simulink model "DigitBreak"  (R2014a)
settings: Solver=FixedStepDiscrete  StartTime=0.0  StopTime=2  FixedStep=1/8000  RelTol=1e-3
undefined symbols (not defined in the file): i
libraries: dspmtrx3 x7, dspsrcs4 x7, simulink x2, dspstat3 x1
settings Model: Creator=Dolby  LastModifiedBy=100432553
settings DataIOCC: SaveOutput=off  SaveTime=off
settings DebuggingCC: UnderspecifiedInitializationDetection=Classic  StateNameClashWarn=warning

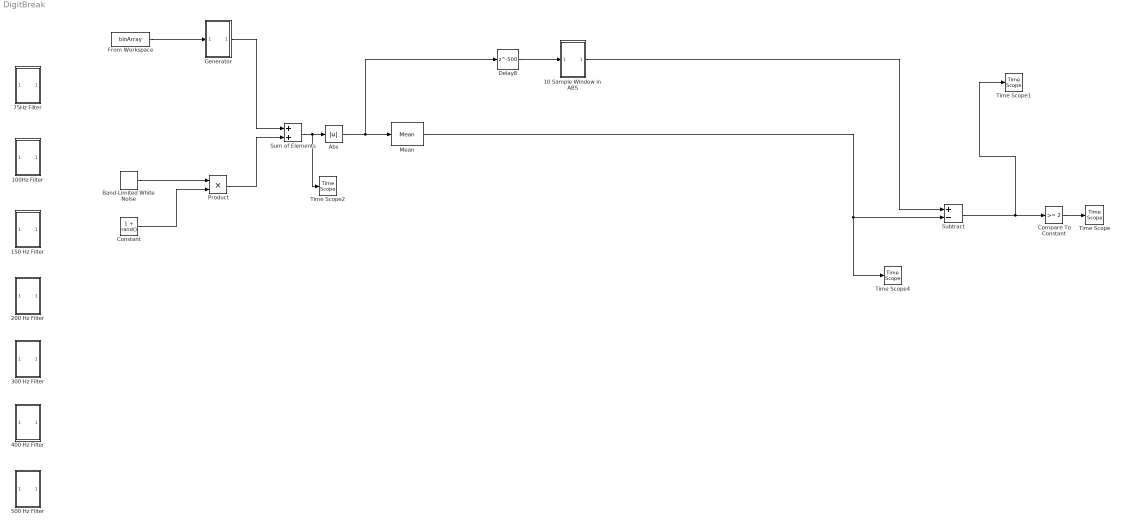
== system DigitBreak ==
  10 Sample Window in ABS : Subsystem
  100Hz Filter : Subsystem
  150 Hz Filter : Subsystem
  200 Hz Filter : Subsystem
  "300 Hz Filter " : Subsystem
  400 Hz Filter : Subsystem
  500 Hz Filter : Subsystem
  75Hz Filter : Subsystem
  Abs : Abs
  Band-Limited White Noise : simulink/Sources/Band-Limited White Noise  Cov=[0.0000001]  Ts=1/8000  seed=[1]
  Compare To Constant : simulink/Logic and Bit Operations/Compare To Constant  relop=>=  const=2  OutDataTypeStr=boolean
  Constant : Constant  Value=1 + rand()
  Delay8 : Delay  DelayLength=500  InitialCondition=0
  From Workspace : FromWorkspace  VariableName=binArray
  Generator : Subsystem
  Mean : dspstat3/Mean  run=on  reset_popup=None  InputProcessing=Columns as channels (frame based)  directionMode=Each column  dimension=1  treatSBRowAsCol=on  roiEnable=off  roiType=Rectangles  roiPortion=Entire ROI  roiOutput=Individual statistics for each ROI  roiFlag=off  outputDataTypeStr=Inherit: Same as accumulator  outputLastDataTypeStr=Inherit: Same as accumulator  outputMin=[]  outputMax=[]  roundingMode=Floor  overflowMode=off
  Product : Product
  Subtract : Sum  Inputs=+-
  Sum of Elements : Sum
  Time Scope{,1..2,4} (4 alike) : TimeScope  DefaultConfigurationName=spbscopes.TimeScopeBlockCfg
  wires:
  From Workspace/1 -> Generator/1(In1)
  Band-Limited White Noise/1 -> Product/1
  Constant/1 -> Product/2
  Sum of Elements/1 -> Time Scope2/1, Abs/1
  Product/1 -> Sum of Elements/2
  Abs/1 -> Mean/1, Delay8/1
  Compare To Constant/1 -> Time Scope/1
  Generator/1(Out1) -> Sum of Elements/1
  Delay8/1 -> 10 Sample Window in ABS/1(In1)
  Mean/1 -> Subtract/2, Time Scope4/1
  Subtract/1 -> Time Scope1/1, Compare To Constant/1
  10 Sample Window in ABS/1(Out1) -> Subtract/1

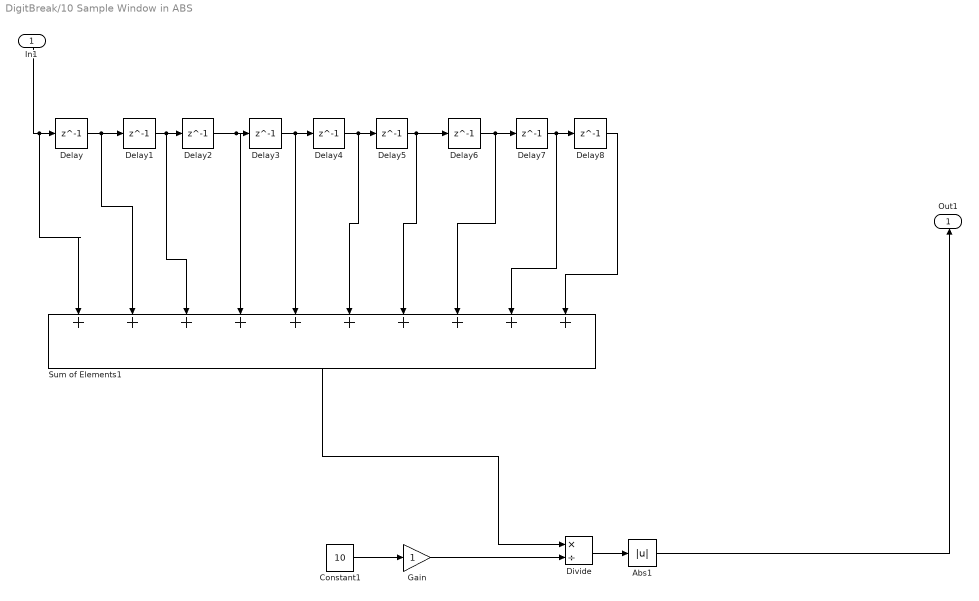
== system DigitBreak/10 Sample Window in ABS ==
  In1 : Inport
  Abs1 : Abs
  Constant1 : Constant  Value=10
  Delay{,1..8} (9 alike) : Delay  DelayLength=1  InitialCondition=0
  Divide : Product  Inputs=*/
  Gain : Gain
  Sum of Elements1 : Sum  Inputs=++++++++++
  Out1 : Outport
  wires:
  Delay4/1 -> Sum of Elements1/6, Delay5/1
  Constant1/1 -> Gain/1
  Divide/1 -> Abs1/1
  Abs1/1 -> Out1/1
  Delay2/1 -> Sum of Elements1/4, Delay3/1
  Delay1/1 -> Sum of Elements1/3, Delay2/1
  Delay/1 -> Sum of Elements1/2, Delay1/1
  Delay3/1 -> Sum of Elements1/5, Delay4/1
  In1/1 -> Delay/1, Sum of Elements1/1
  Gain/1 -> Divide/2
  Sum of Elements1/1 -> Divide/1
  Delay8/1 -> Sum of Elements1/10
  Delay6/1 -> Sum of Elements1/8, Delay7/1
  Delay7/1 -> Sum of Elements1/9, Delay8/1
  Delay5/1 -> Sum of Elements1/7, Delay6/1

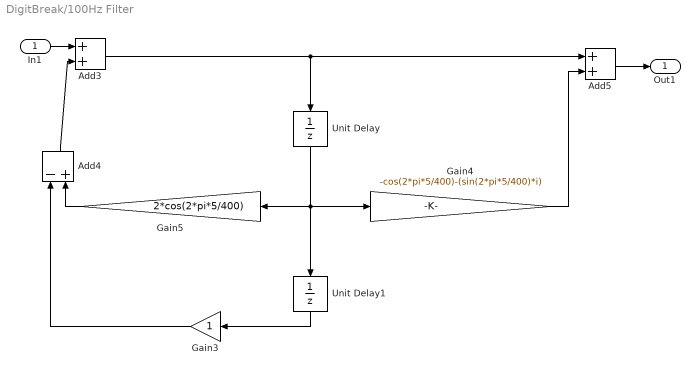
== system DigitBreak/100Hz Filter ==
  In1 : Inport
  Add3 : Sum
  Add4 : Sum  Inputs=-+
  Add5 : Sum
  Gain3 : Gain
  Gain4 : Gain  Gain=-cos(2*pi*5/400)-(sin(2*pi*5/400)*i)
  Gain5 : Gain  Gain=2*cos(2*pi*5/400)
  Unit Delay : UnitDelay  SampleTime=-1
  Unit Delay1 : UnitDelay  SampleTime=-1
  Out1 : Outport
  wires:
  In1/1 -> Add3/1
  Add4/1 -> Add3/2
  Gain3/1 -> Add4/1
  Add3/1 -> Unit Delay/1, Add5/1
  Add5/1 -> Out1/1
  Gain5/1 -> Add4/2
  Gain4/1 -> Add5/2
  Unit Delay1/1 -> Gain3/1
  Unit Delay/1 -> Gain4/1, Unit Delay1/1, Gain5/1

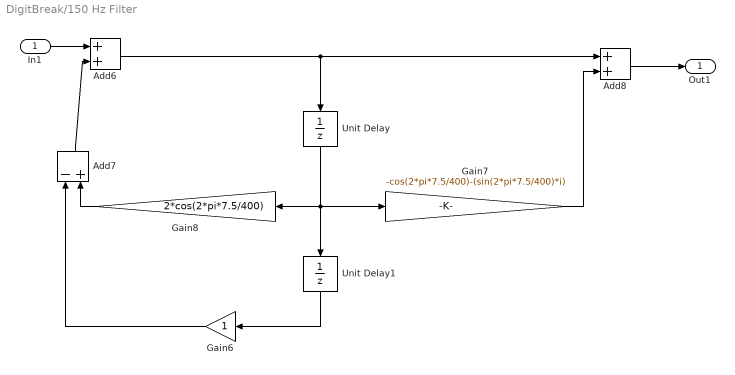
== system DigitBreak/150 Hz Filter ==
  In1 : Inport
  Add6 : Sum
  Add7 : Sum  Inputs=-+
  Add8 : Sum
  Gain6 : Gain
  Gain7 : Gain  Gain=-cos(2*pi*7.5/400)-(sin(2*pi*7.5/400)*i)
  Gain8 : Gain  Gain=2*cos(2*pi*7.5/400)
  Unit Delay : UnitDelay  SampleTime=-1
  Unit Delay1 : UnitDelay  SampleTime=-1
  Out1 : Outport
  wires:
  In1/1 -> Add6/1
  Gain7/1 -> Add8/2
  Add8/1 -> Out1/1
  Gain8/1 -> Add7/2
  Add7/1 -> Add6/2
  Gain6/1 -> Add7/1
  Add6/1 -> Unit Delay/1, Add8/1
  Unit Delay1/1 -> Gain6/1
  Unit Delay/1 -> Gain7/1, Unit Delay1/1, Gain8/1

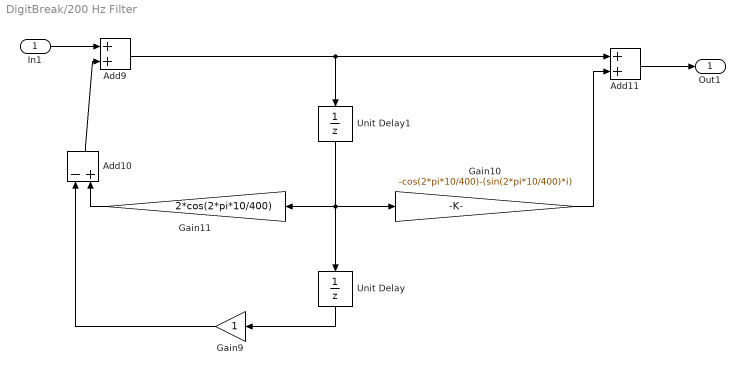
== system DigitBreak/200 Hz Filter ==
  In1 : Inport
  Add10 : Sum  Inputs=-+
  Add11 : Sum
  Add9 : Sum
  Gain10 : Gain  Gain=-cos(2*pi*10/400)-(sin(2*pi*10/400)*i)
  Gain11 : Gain  Gain=2*cos(2*pi*10/400)
  Gain9 : Gain
  Unit Delay : UnitDelay  SampleTime=-1
  Unit Delay1 : UnitDelay  SampleTime=-1
  Out1 : Outport
  wires:
  Gain10/1 -> Add11/2
  Unit Delay1/1 -> Unit Delay/1, Gain10/1, Gain11/1
  Gain9/1 -> Add10/1
  Add10/1 -> Add9/2
  Unit Delay/1 -> Gain9/1
  Add11/1 -> Out1/1
  Add9/1 -> Unit Delay1/1, Add11/1
  Gain11/1 -> Add10/2
  In1/1 -> Add9/1

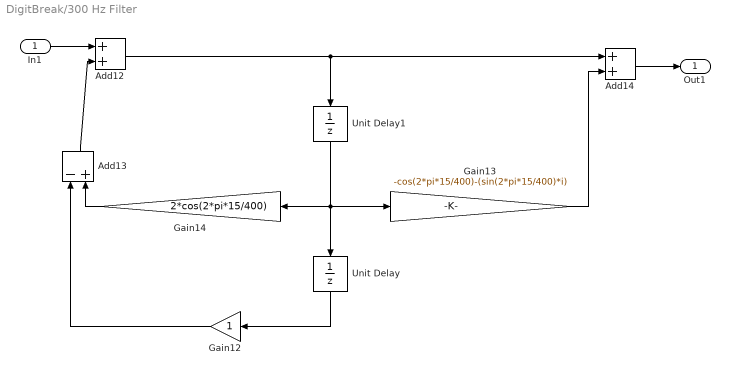
== system DigitBreak/300 Hz Filter  ==
  In1 : Inport
  Add12 : Sum
  Add13 : Sum  Inputs=-+
  Add14 : Sum
  Gain12 : Gain
  Gain13 : Gain  Gain=-cos(2*pi*15/400)-(sin(2*pi*15/400)*i)
  Gain14 : Gain  Gain=2*cos(2*pi*15/400)
  Unit Delay : UnitDelay  SampleTime=-1
  Unit Delay1 : UnitDelay  SampleTime=-1
  Out1 : Outport
  wires:
  Add14/1 -> Out1/1
  Add12/1 -> Unit Delay1/1, Add14/1
  Gain12/1 -> Add13/1
  Unit Delay1/1 -> Unit Delay/1, Gain13/1, Gain14/1
  Add13/1 -> Add12/2
  Gain13/1 -> Add14/2
  Unit Delay/1 -> Gain12/1
  Gain14/1 -> Add13/2
  In1/1 -> Add12/1

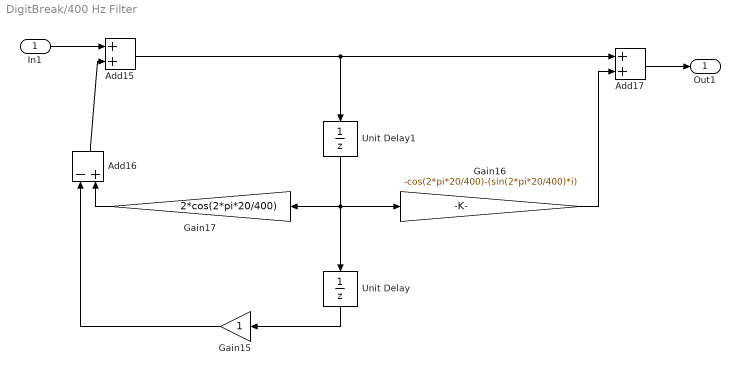
== system DigitBreak/400 Hz Filter ==
  In1 : Inport
  Add15 : Sum
  Add16 : Sum  Inputs=-+
  Add17 : Sum
  Gain15 : Gain
  Gain16 : Gain  Gain=-cos(2*pi*20/400)-(sin(2*pi*20/400)*i)
  Gain17 : Gain  Gain=2*cos(2*pi*20/400)
  Unit Delay : UnitDelay  SampleTime=-1
  Unit Delay1 : UnitDelay  SampleTime=-1
  Out1 : Outport
  wires:
  Gain17/1 -> Add16/2
  Add16/1 -> Add15/2
  Add15/1 -> Unit Delay1/1, Add17/1
  Gain15/1 -> Add16/1
  Unit Delay1/1 -> Gain16/1, Gain17/1, Unit Delay/1
  Gain16/1 -> Add17/2
  Add17/1 -> Out1/1
  Unit Delay/1 -> Gain15/1
  In1/1 -> Add15/1

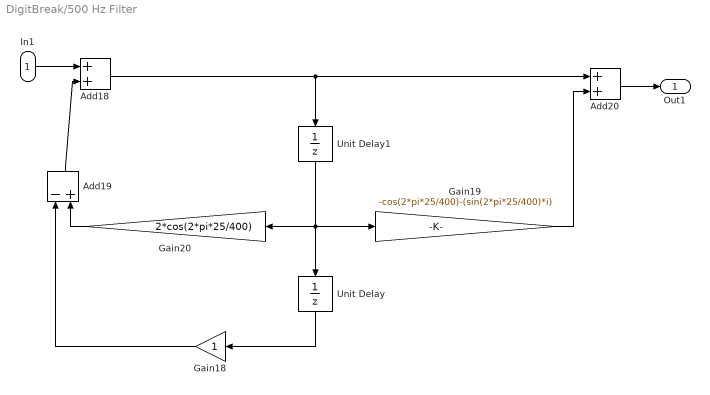
== system DigitBreak/500 Hz Filter ==
  In1 : Inport
  Add18 : Sum
  Add19 : Sum  Inputs=-+
  Add20 : Sum
  Gain18 : Gain
  Gain19 : Gain  Gain=-cos(2*pi*25/400)-(sin(2*pi*25/400)*i)
  Gain20 : Gain  Gain=2*cos(2*pi*25/400)
  Unit Delay : UnitDelay  SampleTime=-1
  Unit Delay1 : UnitDelay  SampleTime=-1
  Out1 : Outport
  wires:
  Unit Delay1/1 -> Unit Delay/1, Gain19/1, Gain20/1
  Add19/1 -> Add18/2
  Add18/1 -> Unit Delay1/1, Add20/1
  Gain18/1 -> Add19/1
  Unit Delay/1 -> Gain18/1
  Add20/1 -> Out1/1
  Gain19/1 -> Add20/2
  Gain20/1 -> Add19/2
  In1/1 -> Add18/1

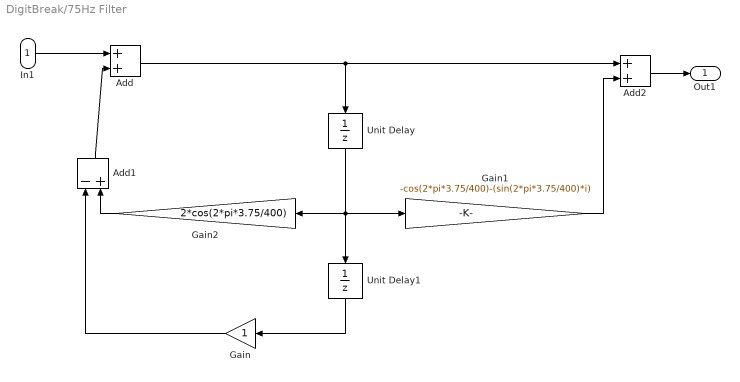
== system DigitBreak/75Hz Filter ==
  In1 : Inport
  Add : Sum  InputSameDT=on
  Add1 : Sum  Inputs=-+
  Add2 : Sum  InputSameDT=on
  Gain : Gain
  Gain1 : Gain  Gain=-cos(2*pi*3.75/400)-(sin(2*pi*3.75/400)*i)
  Gain2 : Gain  Gain=2*cos(2*pi*3.75/400)
  Unit Delay : UnitDelay  SampleTime=-1
  Unit Delay1 : UnitDelay  SampleTime=-1
  Out1 : Outport
  wires:
  In1/1 -> Add/1
  Add2/1 -> Out1/1
  Gain/1 -> Add1/1
  Gain2/1 -> Add1/2
  Gain1/1 -> Add2/2
  Add1/1 -> Add/2
  Add/1 -> Unit Delay/1, Add2/1
  Unit Delay1/1 -> Gain/1
  Unit Delay/1 -> Unit Delay1/1, Gain1/1, Gain2/1

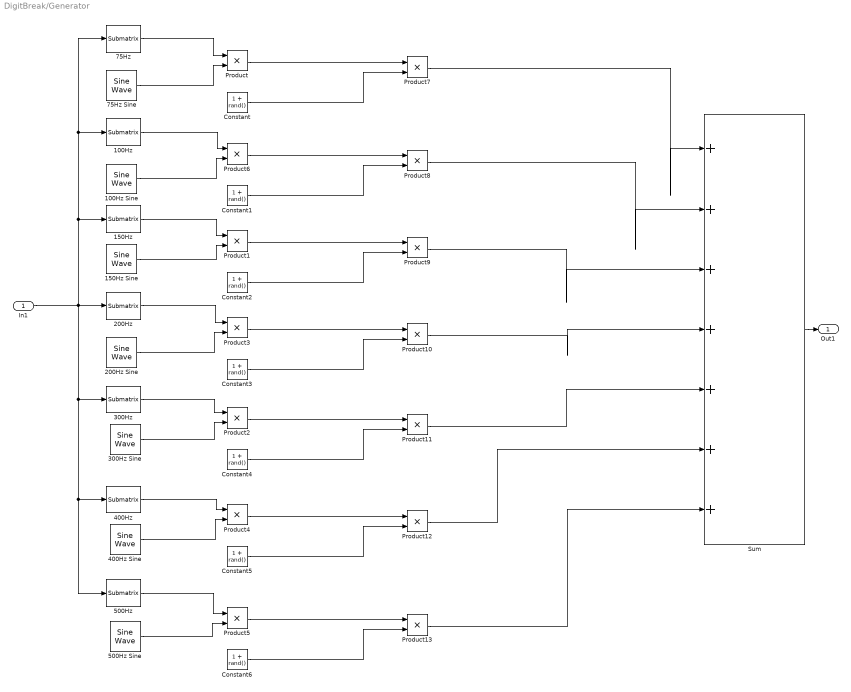
== system DigitBreak/Generator ==
  In1 : Inport
  100Hz : dspmtrx3/Submatrix  RowSpan=One row  RowStartMode=Index  RowStartIndex=2  RowEndMode=Last  RowEndIndex=1  ColSpan=Range of columns  ColStartMode=First  ColStartIndex=1  ColEndMode=Last  ColEndIndex=1
  100Hz Sine : dspsrcs4/Sine Wave  Amplitude=1 + rand()  Frequency=100  Phase=0  SampleMode=Discrete  OutComplex=Real  CompMethod=Trigonometric fcn  TableSize=Speed  SampleTime=1/8000  SamplesPerFrame=1  ResetState=Restart at time zero  dataType=double  wordLen=16  udDataType=sfix(16)  fracBitsMode=Best precision  numFracBits=15  OutDataTypeStr=double  LastOutDataTypeStr=double
  150Hz : dspmtrx3/Submatrix  RowSpan=One row  RowStartMode=Index  RowStartIndex=3  RowEndMode=Last  RowEndIndex=1  ColSpan=Range of columns  ColStartMode=First  ColStartIndex=1  ColEndMode=Last  ColEndIndex=1
  150Hz Sine : dspsrcs4/Sine Wave  Amplitude=1 + rand()  Frequency=150  Phase=0  SampleMode=Discrete  OutComplex=Real  CompMethod=Trigonometric fcn  TableSize=Speed  SampleTime=1/8000  SamplesPerFrame=1  ResetState=Restart at time zero  dataType=double  wordLen=16  udDataType=sfix(16)  fracBitsMode=Best precision  numFracBits=15  OutDataTypeStr=double  LastOutDataTypeStr=double
  200Hz : dspmtrx3/Submatrix  RowSpan=One row  RowStartMode=Index  RowStartIndex=4  RowEndMode=Last  RowEndIndex=1  ColSpan=Range of columns  ColStartMode=First  ColStartIndex=1  ColEndMode=Last  ColEndIndex=1
  200Hz Sine : dspsrcs4/Sine Wave  Amplitude=1 + rand()  Frequency=200  Phase=0  SampleMode=Discrete  OutComplex=Real  CompMethod=Trigonometric fcn  TableSize=Speed  SampleTime=1/8000  SamplesPerFrame=1  ResetState=Restart at time zero  dataType=double  wordLen=16  udDataType=sfix(16)  fracBitsMode=Best precision  numFracBits=15  OutDataTypeStr=double  LastOutDataTypeStr=double
  300Hz : dspmtrx3/Submatrix  RowSpan=One row  RowStartMode=Index  RowStartIndex=5  RowEndMode=Last  RowEndIndex=1  ColSpan=Range of columns  ColStartMode=First  ColStartIndex=1  ColEndMode=Last  ColEndIndex=1
  300Hz Sine : dspsrcs4/Sine Wave  Amplitude=1 + rand()  Frequency=300  Phase=0  SampleMode=Discrete  OutComplex=Real  CompMethod=Trigonometric fcn  TableSize=Speed  SampleTime=1/8000  SamplesPerFrame=1  ResetState=Restart at time zero  dataType=double  wordLen=16  udDataType=sfix(16)  fracBitsMode=Best precision  numFracBits=15  OutDataTypeStr=double  LastOutDataTypeStr=double
  400Hz : dspmtrx3/Submatrix  RowSpan=One row  RowStartMode=Index  RowStartIndex=6  RowEndMode=Last  RowEndIndex=1  ColSpan=Range of columns  ColStartMode=First  ColStartIndex=1  ColEndMode=Last  ColEndIndex=1
  400Hz Sine : dspsrcs4/Sine Wave  Amplitude=1 + rand()  Frequency=200  Phase=0  SampleMode=Discrete  OutComplex=Real  CompMethod=Trigonometric fcn  TableSize=Speed  SampleTime=1/8000  SamplesPerFrame=1  ResetState=Restart at time zero  dataType=double  wordLen=16  udDataType=sfix(16)  fracBitsMode=Best precision  numFracBits=15  OutDataTypeStr=double  LastOutDataTypeStr=double
  500Hz : dspmtrx3/Submatrix  RowSpan=One row  RowStartMode=Last  RowStartIndex=1  RowEndMode=Last  RowEndIndex=1  ColSpan=Range of columns  ColStartMode=First  ColStartIndex=1  ColEndMode=Last  ColEndIndex=1
  500Hz Sine : dspsrcs4/Sine Wave  Amplitude=1 + rand()  Frequency=500  Phase=0  SampleMode=Discrete  OutComplex=Real  CompMethod=Trigonometric fcn  TableSize=Speed  SampleTime=1/8000  SamplesPerFrame=1  ResetState=Restart at time zero  dataType=double  wordLen=16  udDataType=sfix(16)  fracBitsMode=Best precision  numFracBits=15  OutDataTypeStr=double  LastOutDataTypeStr=double
  75Hz : dspmtrx3/Submatrix  RowSpan=One row  RowStartMode=First  RowStartIndex=1  RowEndMode=Last  RowEndIndex=1  ColSpan=Range of columns  ColStartMode=First  ColStartIndex=1  ColEndMode=Last  ColEndIndex=1
  75Hz Sine : dspsrcs4/Sine Wave  Amplitude=1 + rand()  Frequency=75  Phase=0  SampleMode=Discrete  OutComplex=Real  CompMethod=Trigonometric fcn  TableSize=Speed  SampleTime=1/8000  SamplesPerFrame=1  ResetState=Restart at time zero  dataType=double  wordLen=16  udDataType=sfix(16)  fracBitsMode=Best precision  numFracBits=15  OutDataTypeStr=double  LastOutDataTypeStr=double
  Constant{,1..6} (7 alike) : Constant  Value=1 + rand()
  Product{,1..13} (14 alike) : Product
  Sum : Sum  Inputs=|+++++++
  Out1 : Outport
  wires:
  Sum/1 -> Out1/1
  In1/1 -> 200Hz/1, 150Hz/1, 100Hz/1, 75Hz/1, 300Hz/1, 400Hz/1, 500Hz/1
  200Hz Sine/1 -> Product3/2
  400Hz Sine/1 -> Product4/2
  300Hz Sine/1 -> Product2/2
  75Hz Sine/1 -> Product/2
  500Hz Sine/1 -> Product5/2
  150Hz/1 -> Product1/1
  150Hz Sine/1 -> Product1/2
  200Hz/1 -> Product3/1
  100Hz Sine/1 -> Product6/2
  100Hz/1 -> Product6/1
  300Hz/1 -> Product2/1
  75Hz/1 -> Product/1
  400Hz/1 -> Product4/1
  500Hz/1 -> Product5/1
  Product/1 -> Product7/1
  Constant/1 -> Product7/2
  Product6/1 -> Product8/1
  Constant1/1 -> Product8/2
  Product1/1 -> Product9/1
  Constant2/1 -> Product9/2
  Product3/1 -> Product10/1
  Constant3/1 -> Product10/2
  Product2/1 -> Product11/1
  Constant4/1 -> Product11/2
  Product4/1 -> Product12/1
  Constant5/1 -> Product12/2
  Product5/1 -> Product13/1
  Constant6/1 -> Product13/2
  Product13/1 -> Sum/7
  Product12/1 -> Sum/6
  Product11/1 -> Sum/5
  Product10/1 -> Sum/4
  Product9/1 -> Sum/3
  Product8/1 -> Sum/2
  Product7/1 -> Sum/1
